simulink model "On_orbit_satellite_control_basic4"  (R2022a)
settings: Solver=ode4  StartTime=0.0  StopTime=10000  FixedStep=0.1  RelTol=1e-3
libraries: sharedtransform x5, aerolibutil x2, sharedutil x1
settings Model: Creator=sakur  LastModifiedBy=sakur

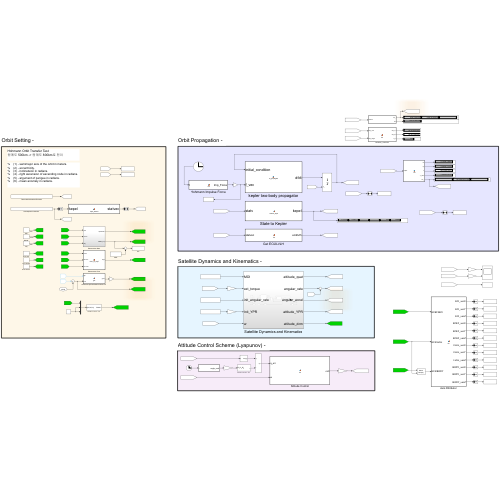
[thumbnail: Simulink's stored preview of the top-level diagram]
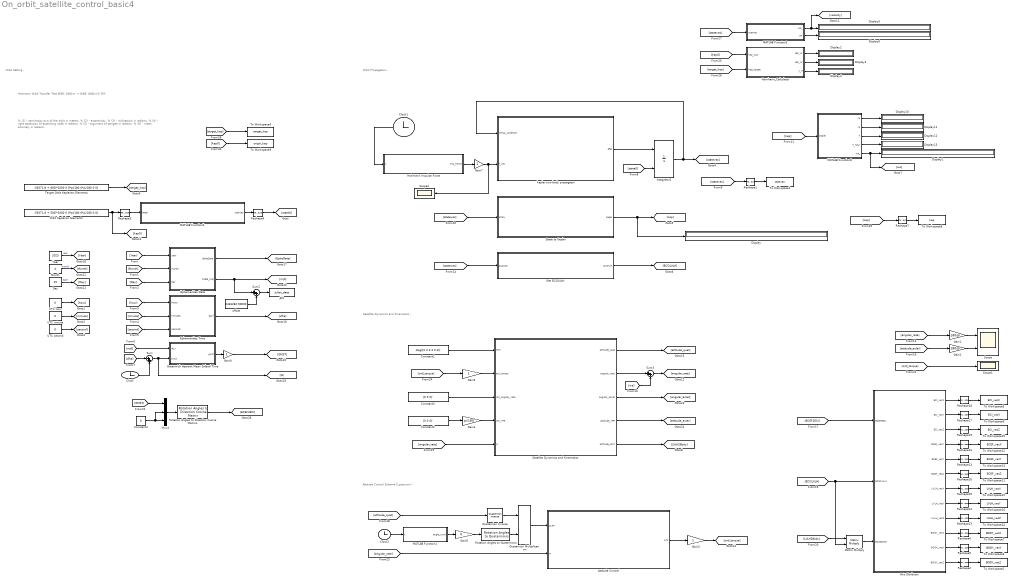
== system On_orbit_satellite_control_basic4 ==
  note: Hohmann Orbit Transfer Test
      | 원궤도 500km -> 원궤도 800km로 전이
  note: Attitude Control Scheme (Lyapunov) -
  note: Satellite Dynamics and Kinematics -
  note: Orbit Setting -
  note: Orbit Propagation -
  note: %		(1) - semimajor axis of the orbit in meters.
      | %		(2) - eccentricity.
      | %		(3) - inclinatsion in radians.
      | %		(4) - right ascension of ascending node in radians.
      | %		(5) - argument of perigee in radians.
      | %		(6) - mean anomaly in radians.
  Attitude Control : MATLAB Function  TreatAsAtomicUnit=on
  Axis Ditributor : MATLAB Function  TreatAsAtomicUnit=on
  Clock : Clock
  Clock1 : Clock
  Clock2 : Clock
  Constant1 : Constant  Value=diag([0.3 0.3 0.3])
  Constant2 : Constant  Value=[0 0 0]'
  Constant3 : Constant  Value=[0 0 0]'
  Constant4 : Constant  Value=0
  Day : Constant  Value=25
  Display{,1..6,10..13} (11 alike) : Display
  Ephemerides Date : Subsystem
  Ephemerides Time : MATLAB Function  TreatAsAtomicUnit=on
  Gain1 : Gain  Gain=180/pi
  Gain2 : Gain  Gain=180/pi
  Gain{3,5,7,9} (4 alike) : Gain
  Gain4 : Gain  Gain=pi/180
  Gain6 : Gain  Gain=0
  Get ECI2LVLH : MATLAB Function  TreatAsAtomicUnit=on
  Greenwich Aparent Mean Sideral Time : MATLAB Function  TreatAsAtomicUnit=on
  Hohmann Impulse Force : MATLAB Function  TreatAsAtomicUnit=on
  Homhann_Calculator : MATLAB Function  TreatAsAtomicUnit=on
  Integrator2 : Integrator  InitialConditionSource=external  InitialCondition=[-7000 0 0 0 -9.175045 0 5233.5]'
  JD1 : ToWorkspace  VariableName=Julian_date  SampleTime=-1
  MATLAB Function1 : MATLAB Function  TreatAsAtomicUnit=on
  MATLAB Function2 : MATLAB Function  TreatAsAtomicUnit=on
  MATLAB Function3 : MATLAB Function  TreatAsAtomicUnit=on
  MATLAB Function8 : MATLAB Function  TreatAsAtomicUnit=on
  Matrix Multiply : Product  Multiplication=Matrix(*)
  Month : Constant  Value=4
  Mux4 : Mux  Inputs=3
  Orbit Keplerian Elements : Constant  Value=[(6371.8 + 500)*1000 0 0*pi/180 0*pi/180 0 0]
  Quaternion Inverse : aerolibutil/Quaternion Inverse
  Quaternion Multiplication : aerolibutil/Quaternion Multiplication
  Reshape{1..7,13,16..19,23..26} (16 alike) : Reshape  OutputDimensionality=Row vector (2-D)
  Rotation Angles to Direction Cosine Matrix1 : sharedtransform/Rotation Angles to Direction Cosine Matrix  rotationOrder=ZYX  aMode=aMode
      settings: SourceProductBaseCode=AE,PW,DR,MT,VE
  Rotation Angles to Quaternions : sharedtransform/Rotation Angles to Quaternions  rotationOrder=ZYX  aMode=aMode
      settings: SourceProductBaseCode=AE,PW,DR,MT,VE
  Satellite Dynamics and Kinematics : Subsystem
  Scope : Scope  NumInputPorts=2
  Scope1 : Scope
  Scope2 : Scope
  State to Kepler : MATLAB Function  TreatAsAtomicUnit=on
  Sum : Sum  Inputs=|++
  Sum2 : Sum  Inputs=|++
  Sum3 : Sum  Inputs=|++
  Target Orbit Keplerian Elements : Constant  Value=[(6371.8 + 800)*1000 0 0*pi/180 0*pi/180 0 0]
  To Workspace1 : ToWorkspace  VariableName=statvec  SampleTime=-1
      settings: Save2DSignal=2-D array (concatenate along first dimension)
  To Workspace10 : ToWorkspace  VariableName=ECI_vecZ  SampleTime=-1
      settings: Save2DSignal=2-D array (concatenate along first dimension)
  To Workspace11 : ToWorkspace  VariableName=ECEF_vecZ  SampleTime=-1
      settings: Save2DSignal=2-D array (concatenate along first dimension)
  To Workspace12 : ToWorkspace  VariableName=ECEF_vecX  SampleTime=-1
      settings: Save2DSignal=2-D array (concatenate along first dimension)
  To Workspace13 : ToWorkspace  VariableName=ECEF_vecY  SampleTime=-1
      settings: Save2DSignal=2-D array (concatenate along first dimension)
  To Workspace14 : ToWorkspace  VariableName=LVLH_vecZ  SampleTime=-1
      settings: Save2DSignal=2-D array (concatenate along first dimension)
  To Workspace15 : ToWorkspace  VariableName=LVLH_vecX  SampleTime=-1
      settings: Save2DSignal=2-D array (concatenate along first dimension)
  To Workspace16 : ToWorkspace  VariableName=LVLH_vecY  SampleTime=-1
      settings: Save2DSignal=2-D array (concatenate along first dimension)
  To Workspace2 : ToWorkspace  VariableName=BODY_vecZ  SampleTime=-1
      settings: Save2DSignal=2-D array (concatenate along first dimension)
  To Workspace3 : ToWorkspace  VariableName=BODY_vecY  SampleTime=-1
      settings: Save2DSignal=2-D array (concatenate along first dimension)
  To Workspace4 : ToWorkspace  VariableName=target_kep  SampleTime=-1
      settings: Save2DSignal=2-D array (concatenate along first dimension)
  To Workspace5 : ToWorkspace  VariableName=ECI_vecX  SampleTime=-1
      settings: Save2DSignal=2-D array (concatenate along first dimension)
  To Workspace6 : ToWorkspace  VariableName=ECI_vecY  SampleTime=-1
      settings: Save2DSignal=2-D array (concatenate along first dimension)
  To Workspace7 : ToWorkspace  VariableName=BODY_vecX  SampleTime=-1
      settings: Save2DSignal=2-D array (concatenate along first dimension)
  To Workspace8 : ToWorkspace  VariableName=kep  SampleTime=-1
      settings: Save2DSignal=2-D array (concatenate along first dimension)
  To Workspace9 : ToWorkspace  VariableName=origin_kep  SampleTime=-1
      settings: Save2DSignal=2-D array (concatenate along first dimension)
  UTC hour : Constant  Value=0
  UTC minute : Constant  Value=0
  UTC second : Constant  Value=0
  Year : Constant  Value=2023
  kepler two-body propagator : MATLAB Function  TreatAsAtomicUnit=on
  offset : Constant  Value=2433282.50000
  wires:
  [cntl_torque] -> Scope1/1
  Matrix Multiply/1 -> Axis Ditributor/3(ECI2BODY)
  Gain9/1 -> [GMST]
  MATLAB Function1/1(angle_cmd) -> Gain6/1
  Satellite Dynamics and Kinematics/5(attitude_dcm) -> [LVLH2Body]
  Gain3/1 -> [cntl_torque]
  MATLAB Function8/3(T) -> Display12/1
  [Day] -> Ephemerides Date/3(day)
  Gain5/1 -> Satellite Dynamics and Kinematics/2(ext_torque)
  [attitude_quat] -> Quaternion Inverse/1
  [cntl_torque] -> Gain5/1
  Ephemerides Date/1(EpheDate) -> [EpheDate]
  Ephemerides Time/1(dayf) -> [dfra]
  [statevec] -> State to Kepler/1(statv)
  [statevec] -> Get ECI2LVLH/1(statvec)
  Clock2/1 -> MATLAB Function1/1(t)
  Attitude Control/1(cntl) -> Gain3/1
  Quaternion Inverse/1 -> Quaternion Multiplication/1
  Quaternion Multiplication/1 -> Attitude Control/1(q_err)
  Axis Ditributor/8(LVLH_vecY) -> Reshape24/1
  Reshape16/1 -> To Workspace12/1
  Reshape18/1 -> To Workspace5/1
  Satellite Dynamics and Kinematics/4(attitude_YPR) -> [attitude_euler]
  Gain2/1 -> Scope/2
  [mjd] -> Greenwich Aparent Mean Sideral Time/1(diju)
  Satellite Dynamics and Kinematics/1(attitude_quat) -> [attitude_quat]
  [angular_rate] -> Attitude Control/2(w)
  Satellite Dynamics and Kinematics/3(angular_accel) -> [angular_accel]
  Axis Ditributor/10(BODY_vecX) -> Reshape6/1
  Axis Ditributor/11(BODY_vecY) -> Reshape5/1
  Constant1/1 -> Satellite Dynamics and Kinematics/1(MOI)
  [dfra] -> Sum/1
  [we] -> Sum3/2
  Sum3/1 -> [angular_rate]
  MATLAB Function8/4(T_hour) -> Display13/1
  Gain4/1 -> Satellite Dynamics and Kinematics/4(Init_YPR)
  Integrator2/1 -> [statevec], kepler two-body propagator/1(initial_condition)
  Gain1/1 -> Scope/1
  UTC hour/1 -> [hour]
  Rotation Angles to Quaternions/1 -> Quaternion Multiplication/2
  [attitude_euler] -> Gain2/1
  Reshape2/1 -> To Workspace2/1
  Clock/1 -> Sum/2
  Reshape26/1 -> To Workspace11/1
  Axis Ditributor/12(BODY_vecZ) -> Reshape2/1
  Month/1 -> [Month]  "month"
  kepler two-body propagator/1(dfdt) -> Integrator2/1
  [ECI2LVLH] -> Matrix Multiply/2, Axis Ditributor/2(ECI2LVLH)
  [statevec] -> Reshape1/1
  Reshape6/1 -> To Workspace7/1
  Reshape19/1 -> To Workspace10/1
  Axis Ditributor/7(LVLH_vecX) -> Reshape25/1
  [state0] -> Integrator2/2
  MATLAB Function8/1(ra) -> Display10/1
  Reshape23/1 -> To Workspace14/1
  offset/1 -> Sum2/2
  [hour] -> Ephemerides Time/1(hours)
  Reshape17/1 -> To Workspace6/1
  [angular_rate] -> Satellite Dynamics and Kinematics/5(w)
  Day/1 -> [Day]  "date"
  Orbit Keplerian Elements/1 -> [kep0], Reshape3/1
  Hohmann Impulse Force/1(Imp_Force) -> Gain7/1
  Sum/1 -> Greenwich Aparent Mean Sideral Time/2(time), [ts]
  Satellite Dynamics and Kinematics/2(angular_rate) -> Sum3/1
  State to Kepler/1(kepel) -> Display/1, [kep]
  Axis Ditributor/3(ECI_vecZ) -> Reshape19/1
  MATLAB Function8/5(we_) -> [we], Display1/1
  [Month] -> Ephemerides Date/2(month)
  Get ECI2LVLH/1(eci2lvlh) -> [ECI2LVLH]
  Rotation Angles to Direction Cosine Matrix1/1 -> [ECEF2ECI]
  Reshape1/1 -> To Workspace1/1
  Reshape25/1 -> To Workspace15/1
  Reshape3/1 -> MATLAB Function2/1(kepel)
  MATLAB Function8/2(rp) -> Display11/1
  Year/1 -> [Year]  "year"
  [angular_rate] -> Gain1/1
  MATLAB Function2/1(statvec) -> Reshape4/1
  Greenwich Aparent Mean Sideral Time/1(gwst) -> Gain9/1
  Axis Ditributor/5(ECEF_vecY) -> Reshape13/1
  Reshape24/1 -> To Workspace16/1
  UTC minute/1 -> [minute]
  [minute] -> Ephemerides Time/2(minutes)
  Constant4/1 -> Mux4/2, Mux4/3
  [GMST] -> Mux4/1
  Mux4/1 -> Rotation Angles to Direction Cosine Matrix1/1
  Constant3/1 -> Satellite Dynamics and Kinematics/3(init_angular_rate)
  [ECEF2ECI] -> Axis Ditributor/1(ECEF2ECI)
  [Year] -> Ephemerides Date/1(year)
  Clock1/1 -> Hohmann Impulse Force/1(t)
  Ephemerides Date/2(CNES_mdj) -> Sum2/1, [mjd]
  UTC second/1 -> [second]
  Axis Ditributor/1(ECI_vecX) -> Reshape18/1
  Axis Ditributor/9(LVLH_vecZ) -> Reshape23/1
  [second] -> Ephemerides Time/3(seconds)
  Axis Ditributor/2(ECI_vecY) -> Reshape17/1
  [LVLH2Body] -> Matrix Multiply/1
  Reshape4/1 -> [state0]
  Constant2/1 -> Gain4/1
  Reshape5/1 -> To Workspace3/1
  [kep] -> MATLAB Function8/1(kepler)
  Axis Ditributor/6(ECEF_vecZ) -> Reshape26/1
  Sum2/1 -> JD1/1
  Reshape13/1 -> To Workspace13/1
  Axis Ditributor/4(ECEF_vecX) -> Reshape16/1
  Target Orbit Keplerian Elements/1 -> [target_kep]
  Gain6/1 -> Rotation Angles to Quaternions/1
  [target_kep] -> Homhann_Calculator/2(kep_target)
  [kep0] -> Homhann_Calculator/1(kep_now)
  Homhann_Calculator/2(del_v2) -> Display3/1
  Homhann_Calculator/1(del_v1) -> Display2/1
  Homhann_Calculator/3(t_H) -> Display4/1
  [statevec] -> MATLAB Function3/1(statvec)
  MATLAB Function3/1(vel_) -> Display5/1, [velocity]
  MATLAB Function3/2(vel) -> Display6/1
  [target_kep] -> To Workspace4/1
  Reshape7/1 -> To Workspace8/1
  [kep] -> Reshape7/1
  Gain7/1 -> Scope2/1, kepler two-body propagator/2(f_vec)
  [kep0] -> To Workspace9/1

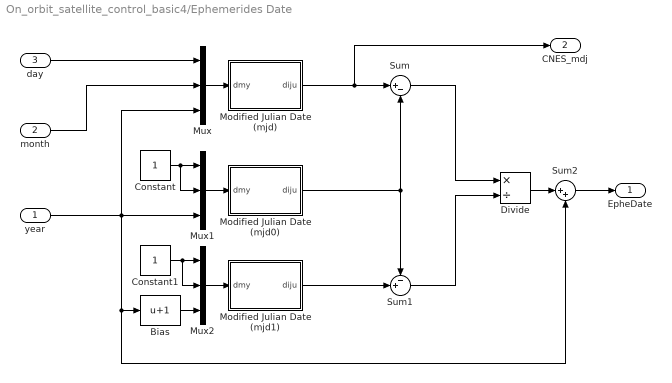
== system On_orbit_satellite_control_basic4/Ephemerides Date ==
  year : Inport
  month : Inport  Port=2
  day : Inport  Port=3
  Bias : Bias  Bias=1  SaturateOnIntegerOverflow=off
  Constant : Constant
  Constant1 : Constant
  Divide : Product  Inputs=*/
  Modified Julian Date (mjd) : MATLAB Function  TreatAsAtomicUnit=on
  Modified Julian Date (mjd0) : MATLAB Function  TreatAsAtomicUnit=on
  Modified Julian Date (mjd1) : MATLAB Function  TreatAsAtomicUnit=on
  Mux : Mux  Inputs=3
  Mux1 : Mux  Inputs=3
  Mux2 : Mux  Inputs=3
  Sum : Sum  Inputs=|+-
  Sum1 : Sum  Inputs=-+|
  Sum2 : Sum  Inputs=|++
  EpheDate : Outport
  CNES_mdj : Outport  Port=2
  wires:
  Sum1/1 -> Divide/2
  Modified Julian Date (mjd1)/1(diju) -> Sum1/2
  month/1 -> Mux/2
  year/1 -> Mux1/3, Mux/3, Bias/1, Sum2/2
  Mux1/1 -> Modified Julian Date (mjd0)/1(dmy)
  day/1 -> Mux/1
  Mux/1 -> Modified Julian Date (mjd)/1(dmy)
  Mux2/1 -> Modified Julian Date (mjd1)/1(dmy)
  Bias/1 -> Mux2/3
  Modified Julian Date (mjd)/1(diju) -> CNES_mdj/1, Sum/1
  Constant1/1 -> Mux2/2, Mux2/1
  Sum/1 -> Divide/1
  Constant/1 -> Mux1/2, Mux1/1
  Modified Julian Date (mjd0)/1(diju) -> Sum1/1, Sum/2
  Divide/1 -> Sum2/1
  Sum2/1 -> EpheDate/1

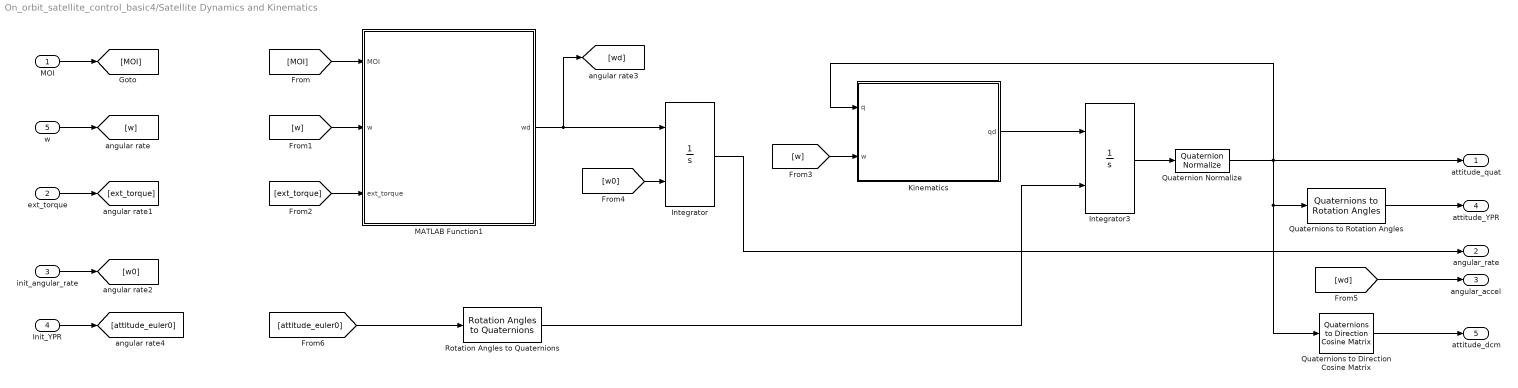
== system On_orbit_satellite_control_basic4/Satellite Dynamics and Kinematics ==
  MOI : Inport
  ext_torque : Inport  Port=2
  init_angular_rate : Inport  Port=3
  Init_YPR : Inport  Port=4
  w : Inport  Port=5
  Integrator : Integrator  InitialConditionSource=external
  Integrator3 : Integrator  InitialConditionSource=external
  Kinematics : MATLAB Function  TreatAsAtomicUnit=on
  MATLAB Function1 : MATLAB Function  TreatAsAtomicUnit=on
  Quaternion Normalize : sharedutil/Quaternion Normalize  aMode=aMode
      settings: SourceProductBaseCode=AE,PW,DR,MT,VE
  Quaternions to Direction Cosine Matrix : sharedtransform/Quaternions to  Direction Cosine Matrix  aMode=aMode
      settings: SourceProductBaseCode=AE,PW,DR,MT,VE
  Quaternions to Rotation Angles : sharedtransform/Quaternions to Rotation Angles  rotationOrder=ZYX  aMode=aMode
      settings: SourceProductBaseCode=AE,PW,DR,MT,VE
  Rotation Angles to Quaternions : sharedtransform/Rotation Angles to Quaternions  rotationOrder=ZYX  aMode=aMode
      settings: SourceProductBaseCode=AE,PW,DR,MT,VE
  attitude_quat : Outport
  angular_rate : Outport  Port=2
  angular_accel : Outport  Port=3
  attitude_YPR : Outport  Port=4
  attitude_dcm : Outport  Port=5
  wires:
  Kinematics/1(qd) -> Integrator3/1
  Quaternion Normalize/1 -> Kinematics/1(q), attitude_quat/1, Quaternions to Direction Cosine Matrix/1, Quaternions to Rotation Angles/1
  Rotation Angles to Quaternions/1 -> Integrator3/2
  Integrator3/1 -> Quaternion Normalize/1
  MATLAB Function1/1(wd) -> [wd], Integrator/1
  Quaternions to Rotation Angles/1 -> attitude_YPR/1
  Quaternions to Direction Cosine Matrix/1 -> attitude_dcm/1
  Integrator/1 -> angular_rate/1
  MOI/1 -> [MOI]
  [MOI] -> MATLAB Function1/1(MOI)
  w/1 -> [w]
  ext_torque/1 -> [ext_torque]
  [w] -> MATLAB Function1/2(w)
  [ext_torque] -> MATLAB Function1/3(ext_torque)
  [w] -> Kinematics/2(w)
  init_angular_rate/1 -> [w0]
  [w0] -> Integrator/2
  [wd] -> angular_accel/1
  Init_YPR/1 -> [attitude_euler0]
  [attitude_euler0] -> Rotation Angles to Quaternions/1

== matlab function On_orbit_satellite_control_basic4/Ephemerides Date/Modified Julian Date (mjd) ==
  data: dmy input; diju output
function diju  =  djm (dmy)
% [diju] = djm (day, month, year)
%    The function djm furnishes the Modified Julian
%    Date with reference to the day, month and year,
%    at zero hours of the day.
% inputs:
%   dmy(1): day, day of the month
%   dmy(2): month, month of the year
%   dmy(3): year

% outputs:
%   diju
%       Modified Julian Date in days, referred to 1950.0. 
%
% Valdemir Carrara, Apr, 2003
%

diju = 367*dmy(3) + dmy(1) - 712269 + fix(275*dmy(2)/9)- fix(7*(dmy(3)+fix((dmy(2)+9)/12))/4);

== matlab function On_orbit_satellite_control_basic4/Axis Ditributor ==
  data: ECEF2ECI input; ECI_vecX output; ECI_vecY output; ECI_vecZ output; ECEF_vecX output; ECEF_vecY output; ECEF_vecZ output; LVLH_vecX output; LVLH_vecY output; LVLH_vecZ output; ECI2LVLH input; ECI2BODY input; BODY_vecX output; BODY_vecY output; BODY_vecZ output
function [ ECI_vecX,  ECI_vecY,  ECI_vecZ,...
          ECEF_vecX, ECEF_vecY, ECEF_vecZ,...
          LVLH_vecX, LVLH_vecY, LVLH_vecZ,...
          BODY_vecX, BODY_vecY, BODY_vecZ] = ...
          fcn(ECEF2ECI, ECI2LVLH, ECI2BODY)

ECI_vecX  = [5000000, 0, 0]';
ECI_vecY  = [0, 5000000, 0]';
ECI_vecZ  = [0, 0, 5000000]';

ECEF_vecX = ECEF2ECI'*ECI_vecX;
ECEF_vecY = ECEF2ECI'*ECI_vecY;
ECEF_vecZ = ECEF2ECI'*ECI_vecZ;

sc=0.5;
LVLH_vecX = ECI2LVLH'*ECI_vecX*sc;
LVLH_vecY = ECI2LVLH'*ECI_vecY*sc;
LVLH_vecZ = ECI2LVLH'*ECI_vecZ*sc;

BODY_vecX = ECI2BODY'*ECI_vecX*sc;
BODY_vecY = ECI2BODY'*ECI_vecY*sc;
BODY_vecZ = ECI2BODY'*ECI_vecZ*sc;
% BODY_vecX = LVLH2BODY(:,1)*500000;
% BODY_vecY = LVLH2BODY(:,2)*500000;
% BODY_vecZ = LVLH2BODY(:,3)*500000;


end

== matlab function On_orbit_satellite_control_basic4/Ephemerides Date/Modified Julian Date (mjd0) ==
  data: dmy input; diju output
function diju  =  djm (dmy)
% [diju] = djm (day, month, year)
%    The function djm furnishes the Modified Julian
%    Date with reference to the day, month and year,
%    at zero hours of the day.
% inputs:
%   dmy(1): day, day of the month
%   dmy(2): month, month of the year
%   dmy(3): year

% outputs:
%   diju
%       Modified Julian Date in days, referred to 1950.0. 
%
% Valdemir Carrara, Apr, 2003
%

diju = 367*dmy(3) + dmy(1) - 712269 + fix(275*dmy(2)/9)- fix(7*(dmy(3)+fix((dmy(2)+9)/12))/4);

== matlab function On_orbit_satellite_control_basic4/Ephemerides Date/Modified Julian Date (mjd1) ==
  data: dmy input; diju output
function diju  =  djm (dmy)
% [diju] = djm (day, month, year)
%    The function djm furnishes the Modified Julian
%    Date with reference to the day, month and year,
%    at zero hours of the day.
% inputs:
%   dmy(1): day, day of the month
%   dmy(2): month, month of the year
%   dmy(3): year

% outputs:
%   diju
%       Modified Julian Date in days, referred to 1950.0. 
%
% Valdemir Carrara, Apr, 2003
%

diju = 367*dmy(3) + dmy(1) - 712269 + fix(275*dmy(2)/9)- fix(7*(dmy(3)+fix((dmy(2)+9)/12))/4);

== matlab function On_orbit_satellite_control_basic4/Ephemerides Time ==
  data: hours input; dayf output; minutes input; seconds input
function dayf  = time_to_dayf(hours, minutes, seconds)
% [dayf] = time_to_dayf (hours, minutes, seconds)
%    The function time_to_dayf returns with the day elapesed
%    time in seconds
% inputs:
%   hours     
%       day hour (integer).
%   minutes
%       minutes (integer).
%   seconds
%       seconds and fraction of second
% outputs:
%   dayf
%       Day elapsed time in seconds. 
%
% Valdemir Carrara, Feb, 2009
%

dayf = seconds + 60*(minutes + 60*hours);

== matlab function On_orbit_satellite_control_basic4/MATLAB Function8 ==
  data: kepler input; ra output; rp output; T output; T_hour output; we_ output
function [ra, rp, T, T_hour, we_] = fcn(kepler)

u=3.9865*10^14;

a = kepler(1);
e = kepler(2);
% 

ra = a*(1+e);%장반경
rp = a*(1-e);%단반경

a = (ra+rp)/2;% semi-major axis

% a = (550 + 6371.8)*1000;

T = 2*pi*sqrt((a*a*a)/(u));% 1 궤도 주기

T_hour = T/3600;

we = 2*pi/T;

we_ = [0 we 0]';%LVLH frame에서 y축이 궤도와 수직함, 즉 y축이 곧 회전축이라 이러헥 정의

end

== matlab function On_orbit_satellite_control_basic4/Satellite Dynamics and Kinematics/Kinematics ==
  data: q input; qd output; w input
function qd    = kinematics( q, w )
w1 = w(1);  w2 = w(2);  w3 = w(3);

Omega = [ 0 -w1 -w2 -w3; 
         w1   0  w3 -w2;
         w2 -w3   0  w1;
         w3  w2 -w1   0];

qd = 0.5*Omega*q;


end

== matlab function On_orbit_satellite_control_basic4/Get ECI2LVLH ==
  data: statvec input; eci2lvlh output
function eci2lvlh  = fcn(statvec)
r = statvec(1:3)';% wrt eci
v = statvec(4:6)';% wrt eci

LVLH_Z = -r/norm(r);
LVLH_Y = -cross(v,LVLH_Z)/norm(cross(v,LVLH_Z));
LVLH_X =  cross(LVLH_Y, LVLH_Z);

eci2lvlh = [LVLH_X,LVLH_Y,LVLH_Z]';

end

== matlab function On_orbit_satellite_control_basic4/Satellite Dynamics and Kinematics/MATLAB Function1 ==
  data: MOI input; wd output; w input; ext_torque input
function wd = Dynamics(MOI, w, ext_torque)

wd = inv(MOI)*(ext_torque - cross(w, MOI*w));

end

== matlab function On_orbit_satellite_control_basic4/kepler two-body propagator ==
  data: initial_condition input; dfdt output; f_vec input
function dfdt  = eq_propagate(initial_condition, f_vec)

u  = 3.9865*10^14;
Re = 6378137; % earth radius in m
sat_mass = 100;%[kg]

dfdt = zeros(size(initial_condition));

x1 = initial_condition(4); % x1 = dx/dt
y1 = initial_condition(5); % y1 = dy/dt
z1 = initial_condition(6); % z1 = dz/dt
x  = initial_condition(1); % x
y  = initial_condition(2); % y
z  = initial_condition(3); % z

r=sqrt(x^2+y^2+z^2);

% % %   Keplar Motion Equatnion
% % %  => r_dd + u/(r^3)r_ = 0 => r_dd = -u/(r^3)r_
dfdt(1) = x1;
dfdt(2) = y1;
dfdt(3) = z1;
dfdt(4) = -u*x/r^3 + f_vec(1)/sat_mass;
dfdt(5) = -u*y/r^3 + f_vec(2)/sat_mass;
dfdt(6) = -u*z/r^3 + f_vec(3)/sat_mass;

end

== matlab function On_orbit_satellite_control_basic4/MATLAB Function2 ==
  data: kepel input; statvec output
function statvec  = kepel_statvec (kepel)
%  [statvec] = kepel_statvec (kepel)
%	The function kepel_statvec transforms the keplerian
%	elements kepel into the corresponding state vector in
%	the same reference system.
%
% Input:
%	kepel
% 		vector containing the keplerian elements:
%		(1) - semimajor axis of the orbit in meters.
%		(2) - eccentricity.
%		(3) - inclinatsion in radians.
%		(4) - right ascension of ascending node in radians.
%		(5) - argument of perigee in radians.
%		(6) - mean anomaly in radians.
% Output:
%	statvec
%  		state vector in meters and meters/second.
%
% Authors:
%	Helio K. Kuga;
%	Valder M. Medeiros;
%	Valdemir Carrara		february/80		version 1.0
%	Valdemir Carrara		july 2005		(C version)
%   Valdemir Carrara            March/09        Matlab

EARTH_GRAVITY	= 3.9860064e+14;		% Earth's gravitational constant (m**3/s**2)

a    = kepel(1);	% semi-major axis
exc  = kepel(2);	% eccentricity

c1   = sqrt(1. - exc*exc);

%     rotation matrix

orb2iner = rotmaz(-kepel(4))*rotmax(-kepel(3))*rotmaz(-kepel(5));

%     Kepler's equation

E    = kepler(kepel(6), exc);

sE   = sin(E);
cE   = cos(E);
c3   = sqrt(EARTH_GRAVITY/a)/(1. - exc*cE);

%     state vector

statvec = [[a*(cE - exc), a*c1*sE, 0]*orb2iner', [-c3*sE, c1*c3*cE, 0]*orb2iner'];

end

function [rot_mat] = rotmax (angle)
% [rot_mat] = rotmax (angle)
%   To obtain the rotation matrix around the X axis given the
%   rotation angle.
% inputs:
%   angle
%       rotation angle, in radians.
% outputs:
%   rot_mat
%       rotation matrix (3, 3)
%

% Valdemir Carrara, Sep, 1998

coan    =  cos(angle);
sian    =  sin(angle);

rot_mat =  [1, 0, 0; 0, coan, sian; 0, -sian, coan];

end

function [rot_mat] = rotmay (angle)
% [rot_mat] = rotmay (angle)
%   To obtain the rotation matrix around the Y axis given the
%   rotation angle.
% inputs:
%   angle
%       rotation angle, in radians.
% outputs:
%   rot_mat
%       rotation matrix (3, 3)
%

% Valdemir Carrara, Sep, 1998


coan    =  cos(angle);
sian    =  sin(angle);

rot_mat =  [coan, 0, -sian; 0, 1, 0; sian, 0, coan];

end

function [rot_mat] = rotmaz (angle)
% [rot_mat] = rotmaz (angle)
%   To obtain the rotation matrix around the Z axis given the
%   rotation angle.
% inputs:
%   angle
%       rotation angle, in radians.
% outputs:
%   rot_mat
%       rotation matrix (3, 3)
%

% Valdemir Carrara, Sep, 1998

coan    =  cos(angle);
sian    =  sin(angle);

rot_mat =  [coan, sian, 0; -sian, coan, 0; 0, 0, 1];
end

function [eccentric] = kepler (mean_anomaly, eccentricity)
% [eccentric] = kepler (mean_anomaly, eccentricity)
%	The subroutine kepler finds a solution to the
%	kepler's equation.
%
% Input:
%	mean_anomaly
%		mean anomaly in radians.
%	eccentricity
%		eccentricity.
%
% Output:
%	eccentric
%		eccentric anomaly in radians.
%
% Authors:
%	Valder M. de Medeiros		june/81		version 2.0
%	Valdemir Carrara			july 2005	(C version)
%   Valdemir Carrara            March/09        Matlab

exc2    = eccentricity*eccentricity;
am1     = mod (mean_anomaly, 2*pi);
am2     = am1 + am1;
am3     = am1 + am2;
shoot   = am1 + eccentricity*(1. - 0.125*exc2)*sin(am1) + ...
		0.5*exc2*(sin(am2) + 0.75*eccentricity*sin(am3));
shoot   = mod (shoot, 2*pi);

e1      = 1.0;
ic      = 0;

while ((abs(e1) > 1.e-12) && (ic <= 10)) 
	e1    = (shoot - am1 - eccentricity*sin(shoot)) / ...
			(1.0 - eccentricity*cos(shoot));
    shoot = shoot - e1;
    ic    = ic + 1;
end

if (ic >= 10)
    disp ('warning ** subroutine kepler did not converge in 10 iterations');
end

eccentric = shoot;


end

== matlab function On_orbit_satellite_control_basic4/Attitude Control ==
  data: q_err input; cntl output; w input
function cntl = fcn(q_err, w)


qe_w = q_err(  1,1);
qe_v = q_err(2:4,1);

K1 = diag([0.1 0.1 0.1]);
K2 = diag([0.3 0.3 0.3]);

cntl = K1*qe_v - K2*w;

end

== matlab function On_orbit_satellite_control_basic4/Hohmann Impulse Force ==
  settings: updateMethod=DISCRETE
  data: Imp_Force output; t input
function Imp_Force  = fcn(t)

Imp_Force = [0 0 0]';

% % % del v1 = 80.92308...[m/sec]
% % % del v2 = 80.06316...[m/sec]
% % % Transfer Time = 2928 [sec]

if t<1 % 바로 1초동안 ECI 기준 +Y로 가속
%    간단하게 F=ma로 계산
    Imp_Force = [0 80.823*100/1 0]'; %여기서 100은 인공위성 무게[kg]
end

if (t>=2950) && (t<(2950+1)) % 전이시간쯤에 1초동안 다시 ECI기준 -Y로 감속 
%    간단하게 F=ma로 계산
    Imp_Force = [0 -80.063*100/1 0]'; %여기서 100은 인공위성 무게[kg]
end

end

== matlab function On_orbit_satellite_control_basic4/State to Kepler ==
  settings: updateMethod=DISCRETE
  data: statv input; kepel output
function kepel  = statvec_kepel (statv)
%	The function statvec_kepel transforms the state vector statv
%	into the corresponding keplerian elements in the
%	same reference system.
%
% Input:
%	statv
%		state vector in meters and meters/second.
%
% Output:
%	statvec_kepel
%		vector containing the keplerian elements:
%		(1) - semimajor axis of the orbit in meters.
%		(2) - eccentricity.
%		(3) - inclination in radians.
%		(4) - right ascension of ascending node in radians.
%		(5) - argument of perigee in radians.
%		(6) - mean anomaly in radians.

EARTH_GRAVITY	= 3.9860064e+14;		% Earth's gravitational constant (m**3/s**2)

xp     = [statv(1),statv(2),statv(3)];
xv     = [statv(4),statv(5),statv(6)];
r      = sqrt(xp*xp');
vq     = xv*xv';
ainv   = 2.0/(r) - vq/EARTH_GRAVITY;

if ainv <= 0
%     pause(1);
    ainv=0;
end

h      = cross(xp, xv);
hm     = sqrt(h*h');

if (hm < 1.e-10)
    disp (' *** Message from function statvec_kepel: *** ');
    disp (' There are no keplerian elements corresponding to this state vector');
    kepel = [0, 0, 0, 0, 0, 0];
else
    h      = h/hm;
    incl   = acos(h(3));
    raan   = atan2(h(1), -h(2));
    d      = xp*xv' / EARTH_GRAVITY;
    esene  = d * sqrt(EARTH_GRAVITY*ainv);
    ecose  = 1 - r*ainv;
    exc    = sqrt(esene*esene + ecose*ecose);
    E      = atan2(esene, ecose);
    mean   = mod (E - esene, 2*pi);
    an = [0 0 0];
    if mean < 0
        mean = mean + 2*pi;
    end
    if exc < 1.e-10
        arpe = 0;
    else
        dp     = 1./r - ainv;
        ev     = dp*xp - d*xv;
        abev   = sqrt(ev*ev');
        ev     = ev/abev;
        an(1)  = cos(raan);
        an(2)  = sin(raan);
        an(3)  = 0;
        fi     = ev*cross(h, an)';
        arpe = acos(ev*an');
        if fi < 0
            arpe  =  -arpe + 2*pi;
        end
    end

    kepel = [(1./ainv), exc, incl, raan, arpe, mean];
    kepel_save = kepel;
    %         T = 2*pi*sqrt((a*a*a)/(EARTH_GRAVITY));
end


end

== matlab function On_orbit_satellite_control_basic4/MATLAB Function1 ==
  data: t input; angle_cmd output
function angle_cmd = fcn(t)

angle_cmd = [0 0 10*sin(0.01*t)]'*pi/180;%[yaw pitch roll]

end

== matlab function On_orbit_satellite_control_basic4/Homhann_Calculator ==
  data: kep_now input; del_v1 output; kep_target input; del_v2 output; t_H output
function [del_v1, del_v2, t_H] = fcn(kep_now, kep_target)

r1  = kep_now(1);
r2  = kep_target(1);
mu  = 3.9865*10^14;

del_v1 = sqrt(mu/r1)*(sqrt((2*r2)/(r1+r2)) - 1);
del_v2 = sqrt(mu/r2)*(1 - sqrt((2*r1)/(r1+r2)));

r3 = (r1+r2)*(r1+r2)*(r1+r2);

t_H = pi*sqrt(r3/(8*mu));
end

== matlab function On_orbit_satellite_control_basic4/MATLAB Function3 ==
  data: statvec input; vel_ output; vel output
function [vel_, vel] = fcn(statvec)

vel_ = [statvec(4) statvec(5) statvec(6)]';
vel  = norm(vel_);

end

== matlab function On_orbit_satellite_control_basic4/Greenwich Aparent Mean Sideral Time ==
  data: diju input; gwst output; time input
function gwst  = gst (diju, time)
% [gwst] = gst (diju, time)
%   The function gst furnishes the greenwich aparent mean 
%   sidereal time referred to the J2000.0 equator and equinox.
% inputs:
%   diju
%       Modified Julian Date in days, referred to 1950.0.
%   time
%       UT1 time complement in seconds.
% outputs:
%   gwst
%       Greenwich aparent sidereal time in radians
%
% Valdemir Carrara, Apr, 2003
%

tsj = (diju-18262.5)/36525;
tsgo = (24110.54841 + (8640184.812866 + 9.3104e-2*tsj - 6.2e-6*tsj*tsj)*tsj)*pi/43200;
tetp = 7.292116e-5;		% velocidade angular da Terra (rd/s) mean angular velocity of the Earth
gwst = mod(tsgo + time*tetp, 2*pi);
% reference site
% https://www2.mps.mpg.de/homes/fraenz/systems/systems2art/node10.html
%      if (gwst<0) gwst = gwst + 2*pi
